simulink model "qpsk"  (R2025a)
settings: Solver=VariableStepAuto  StartTime=0.0  StopTime=10.0  RelTol=1e-3
libraries: simulink x3, dspfdesign x2, commrandsrc3 x1
settings Model: Creator=thomvs  LastModifiedBy=thomvs

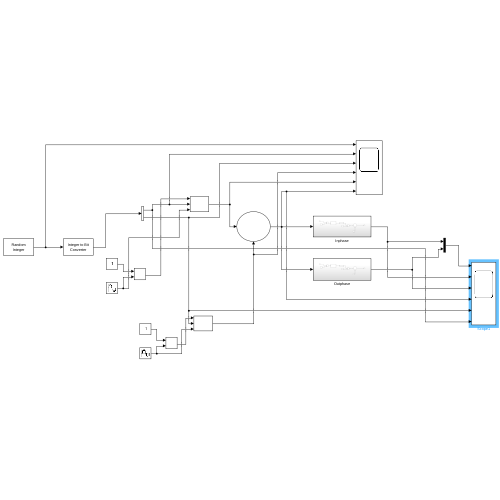
[thumbnail: Simulink's stored preview of the top-level diagram]
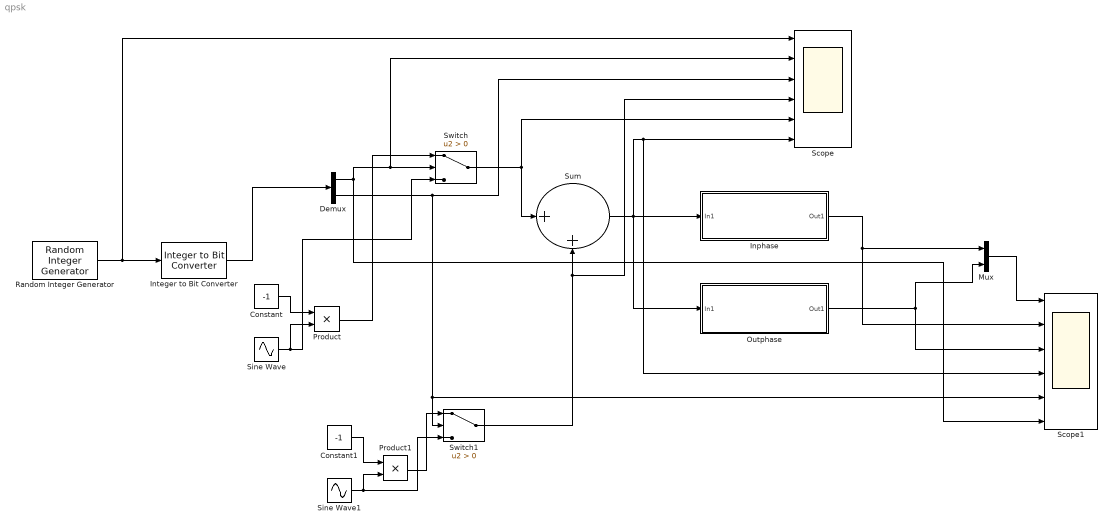
== system qpsk ==
  Constant : Constant  Value=-1
  Constant1 : Constant  Value=-1
  Demux : Demux  Outputs=2
  Inphase : Subsystem
  Integer to Bit Converter : simulink/Logic and Bit Operations/Integer to Bit Converter  nbits=2  signedInputValues=Unsigned  bitOrder=MSB first  outDtype=Inherit via internal rule
  Mux : Mux  Inputs=2
  Outphase : Subsystem
  Product : Product
  Product1 : Product
  Random Integer Generator : commrandsrc3/Random Integer Generator  SetSize=4  SeedSource=Auto  Seed=0  SampleTime=1  SamplesPerFrame=1  OutputDataType=double  SimulateUsing=Interpreted execution
  Scope : Scope  NumInputPorts=6
      settings: ActiveDisplayYMinimum=-0.37499999999999989  ActiveDisplayYMaximum=3.375
  Scope1 : Scope  NumInputPorts=6
      settings: ActiveDisplayYMinimum=-10.635477245372565  ActiveDisplayYMaximum=10.635477245372575
  Sine Wave : Sin  Amplitude=-5  Frequency=2*pi*2  SampleTime=0.01
  Sine Wave1 : Sin  Amplitude=-5  Frequency=2*pi*2  Phase=90  SampleTime=0.01
  Sum : Sum  Inputs=|++
  Switch : Switch  Criteria=u2 > Threshold  SaturateOnIntegerOverflow=off  InputSameDT=off
  Switch1 : Switch  Criteria=u2 > Threshold  SaturateOnIntegerOverflow=off  InputSameDT=off
  wires:
  Random Integer Generator/1 -> Scope/1, Integer to Bit Converter/1
  Constant/1 -> Product/1
  Sine Wave/1 -> Switch/3, Product/2
  Sine Wave1/1 -> Switch1/3, Product1/2
  Constant1/1 -> Product1/1
  Integer to Bit Converter/1 -> Demux/1
  Switch/1 -> Scope/5, Sum/1
  Product/1 -> Switch/1
  Demux/2 -> Scope/3, Switch1/2, Scope1/5
  Product1/1 -> Switch1/1
  Switch1/1 -> Scope/4, Sum/2
  Sum/1 -> Scope1/4, Scope/6, Outphase/1(In1), Inphase/1(In1)
  Demux/1 -> Scope1/6, Scope/2, Switch/2
  Outphase/1(Out1) -> Scope1/3, Mux/2
  Inphase/1(Out1) -> Mux/1, Scope1/2
  Mux/1 -> Scope1/1

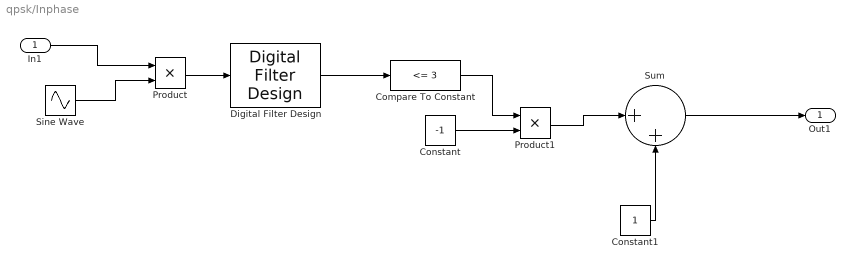
== system qpsk/Inphase ==
  In1 : Inport
  Compare To Constant : simulink/Logic and Bit Operations/Compare To Constant  relop=<=  const=3  OutDataTypeStr=boolean
  Constant : Constant  Value=-1
  Constant1 : Constant
  Digital Filter Design : dspfdesign/Digital Filter Design  mwdsp_browser_bugfix_var=off
  Product : Product
  Product1 : Product
  Sine Wave : Sin  Amplitude=5  Frequency=2*pi*2  SampleTime=0.01
  Sum : Sum  Inputs=|++
  Out1 : Outport
  wires:
  In1/1 -> Product/1
  Sine Wave/1 -> Product/2
  Product/1 -> Digital Filter Design/1
  Digital Filter Design/1 -> Compare To Constant/1
  Constant/1 -> Product1/2
  Compare To Constant/1 -> Product1/1
  Constant1/1 -> Sum/2
  Product1/1 -> Sum/1
  Sum/1 -> Out1/1

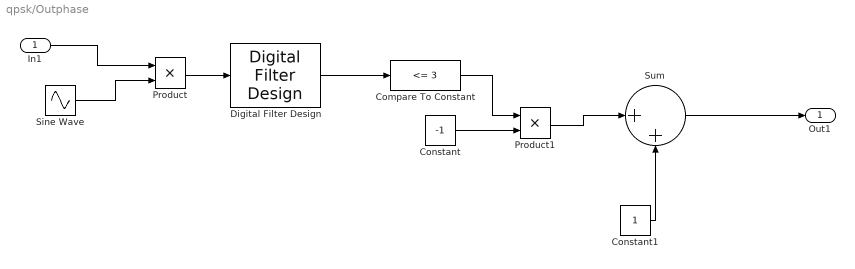
== system qpsk/Outphase ==
  In1 : Inport
  Compare To Constant : simulink/Logic and Bit Operations/Compare To Constant  relop=<=  const=3  OutDataTypeStr=boolean
  Constant : Constant  Value=-1
  Constant1 : Constant
  Digital Filter Design : dspfdesign/Digital Filter Design  mwdsp_browser_bugfix_var=off
  Product : Product
  Product1 : Product
  Sine Wave : Sin  Amplitude=5  Frequency=2*pi*2  Phase=90  SampleTime=0.01
  Sum : Sum  Inputs=|++
  Out1 : Outport
  wires:
  In1/1 -> Product/1
  Sine Wave/1 -> Product/2
  Product/1 -> Digital Filter Design/1
  Digital Filter Design/1 -> Compare To Constant/1
  Constant/1 -> Product1/2
  Compare To Constant/1 -> Product1/1
  Constant1/1 -> Sum/2
  Product1/1 -> Sum/1
  Sum/1 -> Out1/1
